simulink model "dcm_flyback_avg_model_student"  (R2021a)
settings: Solver=ode23tb  StartTime=0.0  StopTime=2  MaxStep=(1/60)/1000  RelTol=1e-4
values from neighbouring files (symbols this model uses):
  C_storage = 2*Pload*t_hold/(V_interm^2 - Vin_min^2)    (= 0.00731645836853)    [final_params.m]
  Cfilt = 1.1e-6    (= 1.1e-06)    [final_params.m]
  D_ss = ( 2 * sqrt((Lmag*Pload)/(Ts)) ) / Vin    [final_params.m]
  freq_in = 60    [final_params.m]
  ki = Gco    (= 10)    [final_params.m]
  kp = (1/wz)*ki    (= 0.76)    [final_params.m]
  Lfilt = 10.2e-3    (= 0.0102)    [final_params.m]
  Lmag = 106e-6    (= 0.000106)    [final_params.m]
  n1 = 2    [final_params.m]
  np = 7    [final_params.m]
  Pload = Pout/eff_target    (= 166.666666667)    [final_params.m]
  Ts = 1/fsw    (= 1e-05)    [final_params.m]
  Vin_rms = 120    [final_params.m]
  Vm = 2    [final_params.m]
  Vref = 2.5    [final_params.m]
undefined symbols (not defined in the file or in its folder): C
libraries: spsVoltageMeasurementLib x6, spsCurrentMeasurementLib x4, spsSeriesRLCBranchLib x4, spsControlledCurrentSourceLib x3, spsControlledVoltageSourceLib x2, spsGroundLib x2, spsRMSLib x2, cstblocks x1, spsMeanLib x1, pid_lib x1, spsTHDLib x1, spsUniversalBridgeLib x1
settings Model: Creator=jvr2131  LastModifiedBy=yoshi
settings SolverCC: ZeroCrossAlgorithm=Adaptive
settings DataIOCC: LimitDataPoints=on  SaveFormat=Array  ReturnWorkspaceOutputs=off
settings OptimizationCC: BlockReduction=off  BooleanDataType=off  LifeSpan=inf
settings DebuggingCC: SaveWithParameterizedLinksMsg=none  UnderspecifiedInitializationDetection=Classic  MergeDetectMultiDrivingBlocksExec=none  SignalResolutionControl=TryResolveAllWithWarning  IgnoredZcDiagnostic=none  MultiTaskDSMMsg=warning  MultiTaskCondExecSysMsg=none  StateNameClashWarn=warning  SFUnexpectedBacktrackingDiag=warning  SFNoUnconditionalDefaultTransitionDiag=warning  SFExecutionAtInitializationDiag=none  SFMachineParentedDataDiag=warning  ArithmeticOperatorsInVariantConditions=warning
settings HardwareCC: ProdBitPerPointer=32  ProdBitPerSizeT=32  ProdBitPerPtrDiffT=32  ProdLargestAtomicFloat=None  ProdIntDivRoundTo=Undefined  ProdEndianess=Unspecified  ProdWordSize=32  ProdHWDeviceType=32-bit Generic  TargetUnknown=on
settings ModelReferenceCC: PropagateSignalLabelsOutOfModel=off
settings SFSimCC: SimUseLocalCustomCode=off  CustomCodeUndefinedFunction=UseInterfaceOnly
settings RTWCC: RTWUseLocalCustomCode=off
settings CodeAppCC: StateflowObjectComments=on
settings GRTTargetCC: TargetLangStandard=C89/C90 (ANSI)
settings ConfigComp: CovMetricSettings=dw  CovSaveCumulativeToWorkspaceVar=on  CovSaveSingleToWorkspaceVar=on  CovExternalEMLEnable=off
settings SimscapeCC: SimscapeNormalizeSystem=off

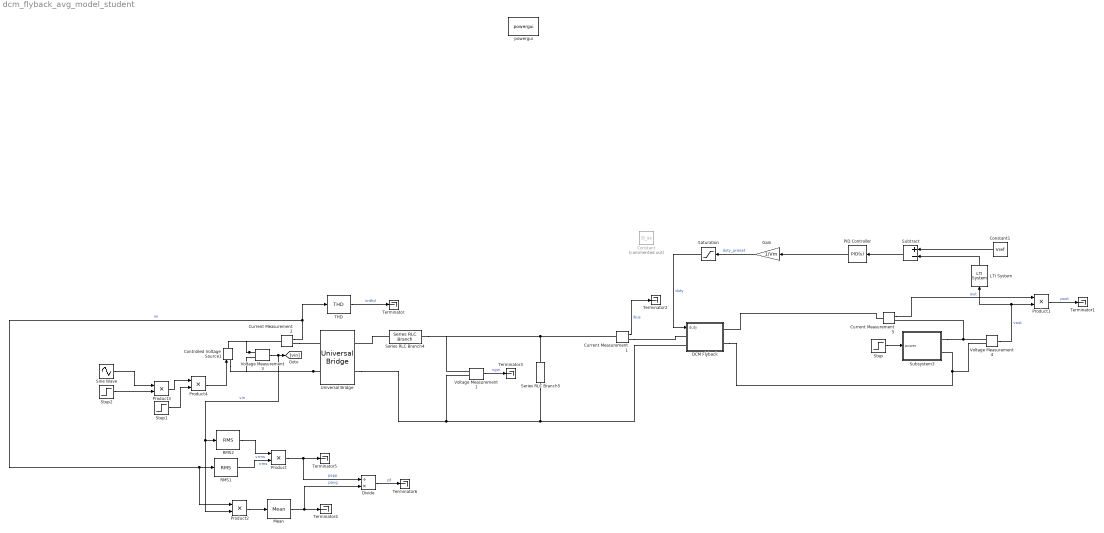
== system dcm_flyback_avg_model_student ==
  Constant : Constant  Commented=on  Value=D_ss
  Constant1 : Constant  Value=Vref
  Controlled Voltage Source1 : spsControlledVoltageSourceLib/Controlled Voltage Source  Initialize=on  Source_Type=AC  Amplitude=0  Phase=0  Frequency=0  Measurements=None
  Current Measurement1 : spsCurrentMeasurementLib/Current Measurement  PhasorSimulation=off  OutputType=Complex  PSBequivalent=0
  Current Measurement2 : spsCurrentMeasurementLib/Current Measurement  PhasorSimulation=off  OutputType=Complex  PSBequivalent=0
  Current Measurement5 : spsCurrentMeasurementLib/Current Measurement  PhasorSimulation=off  OutputType=Complex  PSBequivalent=0
  DCM Flyback : Subsystem
  Divide : Product  Inputs=/*
  Gain : Gain  Gain=1/Vm
  LTI System : cstblocks/LTI System  sys=Htf  IC=[]
  Mean : spsMeanLib/Mean  Freq=60  Vinit=0  Ts=0
  PID Controller : pid_lib/PID Controller  Controller=PID  Form=Parallel  TimeDomain=Continuous-time  UseExternalTs=off  SampleTime=-1  IntegratorMethod=Forward Euler  FilterMethod=Forward Euler  ControllerParametersSource=internal  P=kp  I=ki  D=0  UseFilter=on  N=100  TunerSelectOption=Transfer Function Based (PID Tuner App)  InitialConditionSource=internal  InitialConditionForIntegrator=D_ss*Vm  InitialConditionForFilter=0  DifferentiatorICPrevScaledInput=0  ExternalReset=none  TrackingMode=off  Kt=1  LimitOutput=off  SatLimitsSource=internal  UpperSaturationLimit=inf  LowerSaturationLimit=-inf  LinearizeAsGain=on  AntiWindupMode=none  Kb=1  POutMin=[]  POutMax=[]  IOutMin=[]  IOutMax=[]  DOutMin=[]  DOutMax=[]  NOutMin=[]  NOutMax=[]  SumOutMin=[]  SumOutMax=[]  SaturationOutMin=[]  SaturationOutMax=[]  PParamMin=[]  PParamMax=[]  IParamMin=[]  IParamMax=[]  DParamMin=[]  DParamMax=[]  NParamMin=[]  NParamMax=[]  KbParamMin=[]  KbParamMax=[]  KtParamMin=[]  KtParamMax=[]  KbOutMin=[]  KbOutMax=[]  KtOutMin=[]  KtOutMax=[]  IntegratorOutMin=[]  IntegratorOutMax=[]  FilterOutMin=[]  FilterOutMax=[]  SumI1OutMin=[]  SumI1OutMax=[]  SumI2OutMin=[]  SumI2OutMax=[]  SumI3OutMin=[]  SumI3OutMax=[]  SumI4OutMin=[]  SumI4OutMax=[]  SumDOutMin=[]  SumDOutMax=[]  DifferentiatorOutMin=[]  DifferentiatorOutMax=[]  FilterDiffOutCoefMin=[]  FilterDiffOutCoefMax=[]  ReciprocalOutMin=[]  ReciprocalOutMax=[]  SumDenOutMin=[]  SumDenOutMax=[]  SumNumOutMin=[]  SumNumOutMax=[]  DivideOutMin=[]  DivideOutMax=[]  UdiffTsProdOutMin=[]  UdiffTsProdOutMax=[]  NTsProdOutMin=[]  NTsProdOutMax=[]  UintegralTsProdOutMin=[]  UintegralTsProdOutMax=[]  UngainTsProdOutMin=[]  UngainTsProdOutMax=[]  IntegratorContinuousStateAttributes=''  IntegratorStateMustResolveToSignalObject=off  IntegratorRTWStateStorageClass=Auto  FilterContinuousStateAttributes=''  FilterStateMustResolveToSignalObject=off  FilterRTWStateStorageClass=Auto  ParallelPVariant=InternalParameters  IdealPVariant=Disabled  IVariant=InternalParameters  DVariant=InternalParameters  IntegratorVariant=Continuous  SatVariant=Disabled  AWVariant=Passthrough  PCopyVariant=Disabled  TRVariant=Disabled  FdbkBlocksVariant=Forward  IdealPFdbkVariant=Disabled  SatFdbkVariant=Disabled  DerivativeFilterVariant=ContFilter  NVariant=InternalParameters  NCopyVariant=Disabled  FilterICVariant=InternalICsFilter  IntegratorICVariant=InternalICs  ExternalResetVariant=Disabled  TRSumVariant=Passthrough  SumFdbkVariant=Disabled  SumVariant=Sum_PID  TsampFilterVariant=InternalTs  TsampNgainVariant=Passthrough  TsampIntegralVariant=Passthrough  ExternalSaturationOutDataTypeStr=Inherit: Same as second input
  Product{,1..4} (5 alike) : Product
  RMS1 : spsRMSLib/RMS  TrueRMS=on  Freq=60  RMSInit=120  Ts=0
  RMS2 : spsRMSLib/RMS  TrueRMS=on  Freq=60  RMSInit=120  Ts=0
  Saturation : Saturate  UpperLimit=1  LowerLimit=0
  Series RLC Branch4 : spsSeriesRLCBranchLib/Series RLC Branch  LConnTagsString=__new0  RConnTagsString=__new0  BranchType=L  Resistance=1  Inductance=Lfilt  SetiL0=on  InitialCurrent=0  Capacitance=C  Setx0=on  InitialVoltage=V  Measurements=None
  Series RLC Branch5 : spsSeriesRLCBranchLib/Series RLC Branch  LConnTagsString=__new0  RConnTagsString=__new0  BranchType=C  Resistance=1  Inductance=1e-3  SetiL0=off  InitialCurrent=0  Capacitance=Cfilt  Setx0=on  InitialVoltage=0  Measurements=None
  Sine Wave : Sin  Amplitude=Vin_rms*sqrt(2)  Frequency=2*pi*freq_in  SampleTime=0
  Step : Step  Time=1.2  Before=Pload  After=0.5*Pload  SampleTime=0
  Step1 : Step  Time=0.4333  Before=1  After=100  SampleTime=0
  Step2 : Step  Time=0.4  Before=1  After=0.01  SampleTime=0
  Subsystem3 : Subsystem
  Subtract : Sum  Inputs=+-
  THD : spsTHDLib/THD  Freq=freq_in  Ts=0
      settings: SourceProductBaseCode=PS
  Terminator{,1..6} (7 alike) : Terminator
  Universal Bridge : spsUniversalBridgeLib/Universal Bridge  Arms=2  SnubberResistance=1e5  SnubberCapacitance=inf  Device=Diodes  Ron=1e-3  Lon=0  ForwardVoltages="[  0  0  ]"  ForwardVoltage=0  GTOparameters=[ 10e-6 , 20e-6 ]  IGBTparameters=[ 1e-6 , 2e-6 ]  Measurements=None  Measurements_2=None  converterType=Rectifier
  Voltage Measurement1 : spsVoltageMeasurementLib/Voltage Measurement  PhasorSimulation=off  OutputType=Complex  PSBequivalent=0
  Voltage Measurement3 : spsVoltageMeasurementLib/Voltage Measurement  PhasorSimulation=off  OutputType=Complex  PSBequivalent=0
  Voltage Measurement4 : spsVoltageMeasurementLib/Voltage Measurement  PhasorSimulation=off  OutputType=Complex  PSBequivalent=0
  powergui : spspowerguiLib/powergui  Priority=1  SimulationMode=Continuous  SampleTime=Ts/1000  frequency=60  Iterations=50  frequencyindice=0  Pbase=100e6  ErrMax=1e-4  UnitsV=kV  UnitsW=MW  buscounter=0  FunctionMessages=off  echomessages=off  EnableUseOfTLC=off  CurrentSourceSwitches=off  DisableSnubberDevices=off  DisableRonSwitches=off  DisableVfSwitches=off  DisplayEquations=off  AutomaticDiscreteSolvers=off  SolverType=Tustin/Backward Euler (TBE)  Interpol=off  ExternalGateDelay=off  methode=off  Ts=100  x0status=blocks  SPID=on  SwTol=0  HookPort=off  NonlinearTolerance=1e-4  nMaxIteration=100  ContinueOnMaxIteration=off  RestoreLinks=warning  ResistiveCurrentMeasurement=off  Frange=[0:2:500]  Ylog=off  Xlog=on  ShowGrid=off  save=off  variable=ZData  structure=0  ZoomFFT=off  StartTime=0.0  cycles=1  DisplayStyle=1  fundamental=60  FreqAxis=off  MaxFrequency=1000  frequencyindicesteady=1  RmsSteady=1  display=off
  wires:
  Voltage Measurement3/1 -> Product2/2, RMS2/1, [vin]  "vin"
  Current Measurement2/1 -> RMS1/1, Product2/1, THD/1  "iin"
  THD/1 -> Terminator/1  "iinthd"
  Voltage Measurement4/1 -> Product1/2, LTI System/1  "vout"
  Current Measurement1/1 -> Terminator2/1  "ibus"
  Current Measurement5/1 -> Product1/1  "iout"
  Product1/1 -> Terminator1/1  "pout"
  Step/1 -> Subsystem3/1(power)
  Voltage Measurement1/1 -> Terminator3/1  "vgin"
  Constant1/1 -> Subtract/1
  LTI System/1 -> Subtract/2
  Subtract/1 -> PID Controller/1
  PID Controller/1 -> Gain/1
  RMS2/1 -> Product/1  "vrms"
  Product/1 -> Divide/1, Terminator5/1  "papp"
  Product2/1 -> Mean/1
  Mean/1 -> Divide/2, Terminator4/1  "pavg"
  Divide/1 -> Terminator6/1  "pf"
  RMS1/1 -> Product/2  "irms"
  Step2/1 -> Product3/2
  Sine Wave/1 -> Product3/1
  Step1/1 -> Product4/2
  Product3/1 -> Product4/1
  Product4/1 -> Controlled Voltage Source1/1
  Gain/1 -> Saturation/1  "duty_presat"
  Saturation/1 -> DCM Flyback/1(duty)  "duty"
  connections:
  Universal Bridge/LConn2 -- Voltage Measurement3/LConn2 -- Controlled Voltage Source1/LConn1
  Voltage Measurement3/LConn1 -- Current Measurement2/LConn1 -- Controlled Voltage Source1/RConn1
  Current Measurement2/RConn1 -- Universal Bridge/LConn1
  Universal Bridge/RConn2 -- Series RLC Branch5/RConn1 -- DCM Flyback/LConn2 -- Voltage Measurement1/LConn2
  Subsystem3/RConn1 -- Current Measurement5/RConn1 -- Voltage Measurement4/LConn1
  Current Measurement1/RConn1 -- DCM Flyback/LConn1
  Current Measurement5/LConn1 -- DCM Flyback/RConn1
  Current Measurement1/LConn1 -- Series RLC Branch4/RConn1 -- Voltage Measurement1/LConn1 -- Series RLC Branch5/LConn1
  Series RLC Branch4/LConn1 -- Universal Bridge/RConn1
  Voltage Measurement4/LConn2 -- Subsystem3/RConn2 -- DCM Flyback/RConn2

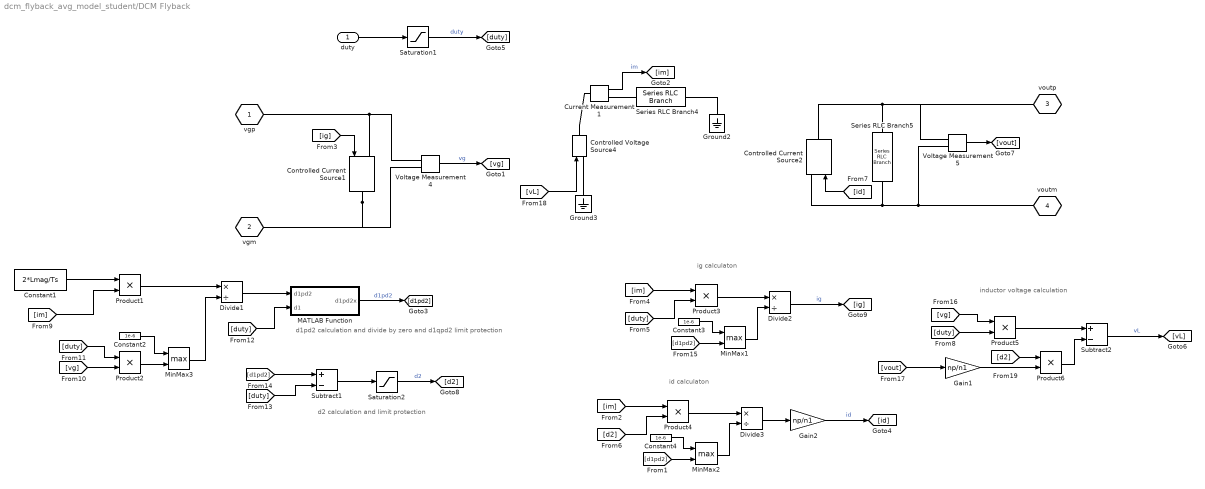
== system dcm_flyback_avg_model_student/DCM Flyback ==
  note: inductor voltage calculation
  note: ig calculaton
  note: d2 calculation and limit protection
  note: d1pd2 calculation and divide by zero and d1qpd2 limit protection
  note: id calculaton
  duty : Inport
  Constant1 : Constant  Value=2*Lmag/Ts
  Constant2 : Constant  Value=1e-6
  Constant3 : Constant  Value=1e-6
  Constant4 : Constant  Value=1e-6
  Controlled Current Source1 : spsControlledCurrentSourceLib/Controlled Current Source  Initialize=on  Source_Type=AC  Amplitude=0  Phase=0  Frequency=0  Measurements=None
  Controlled Current Source2 : spsControlledCurrentSourceLib/Controlled Current Source  Initialize=on  Source_Type=AC  Amplitude=0  Phase=0  Frequency=0  Measurements=None
  Controlled Voltage Source4 : spsControlledVoltageSourceLib/Controlled Voltage Source  Initialize=on  Source_Type=AC  Amplitude=0  Phase=0  Frequency=0  Measurements=None
  Current Measurement1 : spsCurrentMeasurementLib/Current Measurement  PhasorSimulation=off  OutputType=Complex  PSBequivalent=0
  Divide1 : Product  Inputs=*/
  Divide2 : Product  Inputs=*/
  Divide3 : Product  Inputs=*/
  Gain1 : Gain  Gain=np/n1
  Gain2 : Gain  Gain=np/n1
  Ground2 : spsGroundLib/Ground  LConnTagsString=a
  Ground3 : spsGroundLib/Ground  LConnTagsString=a
  MATLAB Function : MATLAB Function  TreatAsAtomicUnit=on
  MinMax1 : MinMax  Function=max  Inputs=2
  MinMax2 : MinMax  Function=max  Inputs=2
  MinMax3 : MinMax  Function=max  Inputs=2
  Product{1..6} (6 alike) : Product
  Saturation1 : Saturate  UpperLimit=1  LowerLimit=0
  Saturation2 : Saturate  UpperLimit=1  LowerLimit=0
  Series RLC Branch4 : spsSeriesRLCBranchLib/Series RLC Branch  LConnTagsString=__new0  RConnTagsString=__new0  BranchType=L  Resistance=1  Inductance=Lmag  SetiL0=off  InitialCurrent=0  Capacitance=C  Setx0=on  InitialVoltage=V  Measurements=None
  Series RLC Branch5 : spsSeriesRLCBranchLib/Series RLC Branch  LConnTagsString=__new0  RConnTagsString=__new0  BranchType=C  Resistance=1  Inductance=1e-3  SetiL0=off  InitialCurrent=0  Capacitance=C_storage  Setx0=on  InitialVoltage=V_interm  Measurements=None
  Subtract1 : Sum  Inputs=+-
  Subtract2 : Sum  Inputs=+-
  Voltage Measurement4 : spsVoltageMeasurementLib/Voltage Measurement  PhasorSimulation=off  OutputType=Complex  PSBequivalent=0
  Voltage Measurement5 : spsVoltageMeasurementLib/Voltage Measurement  PhasorSimulation=off  OutputType=Complex  PSBequivalent=0
  vgp : PMIOPort  Tag=PMCPort  Side=Left
  vgm : PMIOPort  Tag=PMCPort  Port=2  Side=Left
  voutp : PMIOPort  Tag=PMCPort  Port=3  Side=Right
  voutm : PMIOPort  Tag=PMCPort  Port=4  Side=Right
  wires:
  Current Measurement1/1 -> [im]  "im"
  Voltage Measurement5/1 -> [vout]
  duty/1 -> Saturation1/1
  [ig] -> Controlled Current Source1/1
  Voltage Measurement4/1 -> [vg]  "vg"
  Saturation1/1 -> [duty]  "duty"
  Constant1/1 -> Product1/1
  [im] -> Product1/2
  [vg] -> Product2/2
  [duty] -> Product2/1
  Product1/1 -> Divide1/1
  Product2/1 -> MinMax3/2
  MinMax3/1 -> Divide1/2
  Constant2/1 -> MinMax3/1
  [duty] -> MATLAB Function/2(d1)
  Divide1/1 -> MATLAB Function/1(d1pd2)
  MATLAB Function/1(d1pd2x) -> [d1pd2]  "d1pd2"
  [d1pd2] -> Subtract1/1
  [duty] -> Subtract1/2
  Subtract1/1 -> Saturation2/1
  Saturation2/1 -> [d2]  "d2"
  [im] -> Product3/1
  [duty] -> Product3/2
  Product3/1 -> Divide2/1
  [d1pd2] -> MinMax1/2
  MinMax1/1 -> Divide2/2
  Constant3/1 -> MinMax1/1
  Divide2/1 -> [ig]  "ig"
  [d1pd2] -> MinMax2/2
  [d2] -> Product4/2
  MinMax2/1 -> Divide3/2
  Product4/1 -> Divide3/1
  [im] -> Product4/1
  Constant4/1 -> MinMax2/1
  Divide3/1 -> Gain2/1
  Gain2/1 -> [id]  "id"
  [id] -> Controlled Current Source2/1
  [duty] -> Product5/2
  [vg] -> Product5/1
  Product5/1 -> Subtract2/1
  [vout] -> Gain1/1
  Gain1/1 -> Product6/2
  Product6/1 -> Subtract2/2
  Subtract2/1 -> [vL]  "vL"
  [vL] -> Controlled Voltage Source4/1
  [d2] -> Product6/1
  connections:
  Voltage Measurement5/LConn2 -- voutm/RConn1 -- Series RLC Branch5/RConn1 -- Controlled Current Source2/LConn1
  Controlled Current Source1/LConn1 -- vgp/RConn1 -- Voltage Measurement4/LConn1
  Controlled Current Source1/RConn1 -- vgm/RConn1 -- Voltage Measurement4/LConn2
  Ground3/LConn1 -- Controlled Voltage Source4/LConn1
  Current Measurement1/RConn1 -- Series RLC Branch4/LConn1
  Controlled Current Source2/RConn1 -- voutp/RConn1 -- Voltage Measurement5/LConn1 -- Series RLC Branch5/LConn1
  Ground2/LConn1 -- Series RLC Branch4/RConn1
  Controlled Voltage Source4/RConn1 -- Current Measurement1/LConn1

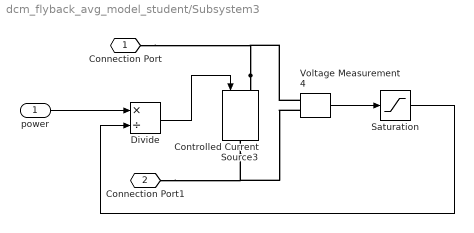
== system dcm_flyback_avg_model_student/Subsystem3 ==
  power : Inport
  Controlled Current Source3 : spsControlledCurrentSourceLib/Controlled Current Source  Initialize=on  Source_Type=AC  Amplitude=0  Phase=0  Frequency=0  Measurements=None
  Divide : Product  Inputs=*/
  Saturation : Saturate  UpperLimit=inf  LowerLimit=1e-3
  Voltage Measurement4 : spsVoltageMeasurementLib/Voltage Measurement  PhasorSimulation=off  OutputType=Complex  PSBequivalent=0
  Connection Port : PMIOPort  Side=Right
  Connection Port1 : PMIOPort  Port=2  Side=Right
  wires:
  Saturation/1 -> Divide/2
  power/1 -> Divide/1
  Voltage Measurement4/1 -> Saturation/1
  Divide/1 -> Controlled Current Source3/1
  connections:
  Controlled Current Source3/RConn1 -- Connection Port1/RConn1 -- Voltage Measurement4/LConn2
  Controlled Current Source3/LConn1 -- Connection Port/RConn1 -- Voltage Measurement4/LConn1

== matlab function dcm_flyback_avg_model_student/DCM Flyback/MATLAB Function ==
  data: d1pd2 input; d1pd2x output; d1 input
function d1pd2x = fcn(d1pd2,d1)

d1pd2x = d1pd2;

if(d1pd2<=d1)
    d1pd2=d1;
end

if(d1pd2>=1)
    d1pd2=1;
end

end
